simulink model "Cruise_Control"  (R2020b)
settings: Solver=VariableStepAuto  StartTime=0.0  StopTime=10.0  RelTol=1e-3
model workspace (MAT data in the model file):
  b = 50
  m = 1000
settings Model: Creator=com  LastModifiedBy=com
settings DataIOCC: SaveOutput=off  SaveTime=off

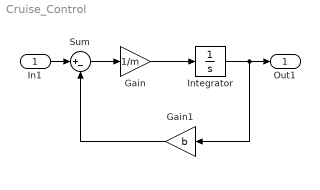
== system Cruise_Control ==
  In1 : Inport  OutDataTypeStr=double  PortDimensions=1  SampleTime=0
  Gain : Gain  Gain=1/m
  Gain1 : Gain  Gain=b
  Integrator : Integrator
  Sum : Sum  Inputs=|+-
  Out1 : Outport  OutDataTypeStr=double  PortDimensions=1  SampleTime=0
  wires:
  Gain1/1 -> Sum/2
  Sum/1 -> Gain/1
  Gain/1 -> Integrator/1
  In1/1 -> Sum/1
  Integrator/1 -> Gain1/1, Out1/1
